simulink model "tp415821"  (Simulink 3.0)
settings: Solver=ode1  SolverMode=SingleTasking  StartTime=0.0  StopTime=t_sim  FixedStep=Ts  RelTol=1e-3
values from neighbouring files (symbols this model uses):
  P = KR    [init_bulb_fan_PI1_disc_windupless.m]
  Ts = 1    [init_bulb_fan_PI1_disc_windupless.m]    (also in prev45_10.mat = 0.2; prev45_2.mat = 0.2; prev45_4.mat = 0.2)
  Umax = 5    [init_bulb_fan_PI1_disc_windupless.m]    (also in prev45_10.mat; prev45_2.mat; prev45_4.mat)
  Umin = -5    [init_bulb_fan_PI1_disc_windupless.m]    (also in prev45_10.mat = 0; prev45_2.mat = 0; prev45_4.mat = 0)
undefined symbols (not defined in the file or in its folder): I
libraries: simulink x1, udaq28LT_lib x1
settings Model: LastModifiedBy=mato  SaveFormat=Matrix  BooleanDataType=on

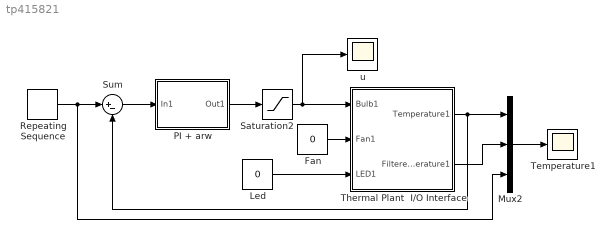
== system tp415821 ==
  Fan : Constant  Value=0
  Led : Constant  Value=0
  Mux2 : Mux  Inputs=3
  PI + arw : Subsystem
  Repeating Sequence : simulink/Sources/Repeating Sequence  rep_seq_t=[0 50 50+Ts 150]  rep_seq_y=[32 32 34 34]
  Saturation2 : Saturate  UpperLimit=Umax  LowerLimit=Umin
  Sum : Sum  Inputs=|+-  SaturateOnIntegerOverflow=on
  Temperature1 : Scope
      settings: TickLabels=on  TimeRange=30  YMin=15  YMax=50  SaveName=yt  DataFormat=Matrix
  Thermal Plant  I/O Interface : Subsystem
      mask Display: disp('Thermo-optical\nPlant\nI/O Interface')
  u : Scope
      settings: TimeRange=150  YMin=-0.5  YMax=5.5  SaveName=u  DataFormat=Matrix  Decimation=10  SampleInput=on  SampleTime=Ts
  wires:
  Saturation2/1 -> u/1, Thermal Plant  I/O Interface/1(Bulb1)
  Sum/1 -> PI + arw/1(In1)
  Repeating Sequence/1 -> Sum/1, Mux2/3
  PI + arw/1(Out1) -> Saturation2/1
  Mux2/1 -> Temperature1/1
  Thermal Plant  I/O Interface/1(Temperature1) -> Mux2/1, Sum/2
  Thermal Plant  I/O Interface/2(Filtered  temperature1) -> Mux2/2
  Fan/1 -> Thermal Plant  I/O Interface/2(Fan1)
  Led/1 -> Thermal Plant  I/O Interface/3(LED1)

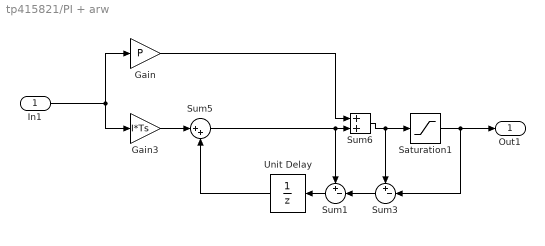
== system tp415821/PI + arw ==
  In1 : Inport  Port=1  PortWidth=-1  SampleTime=-1  DataType=auto
      settings: SignalType=auto
  Gain : Gain  Gain=P  SaturateOnIntegerOverflow=on
  Gain3 : Gain  Gain=I*Ts  SaturateOnIntegerOverflow=on
  Saturation1 : Saturate  UpperLimit=Umax  LowerLimit=Umin
  Sum1 : Sum  Orientation=left  Inputs=+-|  SaturateOnIntegerOverflow=on
  Sum3 : Sum  Orientation=left  Inputs=+-|  SaturateOnIntegerOverflow=on
  Sum5 : Sum  Inputs=|++  SaturateOnIntegerOverflow=on
  Sum6 : Sum  Inputs=++  SaturateOnIntegerOverflow=on
  Unit Delay : UnitDelay  Orientation=left  X0=0  SampleTime=Ts
  Out1 : Outport  Port=1
  wires:
  Sum3/1 -> Sum1/2
  Sum1/1 -> Unit Delay/1
  Gain3/1 -> Sum5/1
  Unit Delay/1 -> Sum5/2
  Sum6/1 -> Sum3/1, Saturation1/1
  Saturation1/1 -> Sum3/2, Out1/1
  In1/1 -> Gain/1, Gain3/1
  Sum5/1 -> Sum1/1, Sum6/2
  Gain/1 -> Sum6/1

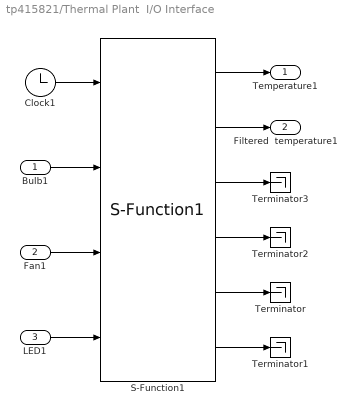
== system tp415821/Thermal Plant  I/O Interface ==
  Bulb1 : Inport  Port=1  PortWidth=-1  SampleTime=-1  DataType=auto
      settings: SignalType=auto
  Fan1 : Inport  Port=2  PortWidth=-1  SampleTime=-1  DataType=auto
      settings: SignalType=auto
  LED1 : Inport  Port=3  PortWidth=-1  SampleTime=-1  DataType=auto
      settings: SignalType=auto
  Clock1 : Clock
      settings: DisplayTime=off  Decimation=10
  S-Function1 : udaq28LT_lib/S-Function1  Priority=1  com_port=COM3  Ts=Ts  events_ot=2  rd_timeout=Ts/2*1000  matlab_prior=ABOVE_NORMAL_PRIORITY  warning=on  printout=off
  Terminator{,1..3} (4 alike) : Terminator
  Temperature1 : Outport  Port=1
  Filtered  temperature1 : Outport  Port=2
  wires:
  S-Function1/1 -> Temperature1/1
  S-Function1/2 -> Filtered  temperature1/1
  Clock1/1 -> S-Function1/1
  Bulb1/1 -> S-Function1/2
  Fan1/1 -> S-Function1/3
  S-Function1/3 -> Terminator3/1
  S-Function1/4 -> Terminator2/1
  S-Function1/5 -> Terminator/1
  S-Function1/6 -> Terminator1/1
  LED1/1 -> S-Function1/4
